simulink model "SFunBinToDes"  (R2019a)
settings: Solver=FixedStepDiscrete  StartTime=0.0  StopTime=10.0  RelTol=1e-3
settings Model: Creator=MY MIND  LastModifiedBy=MY MIND

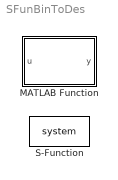
== system SFunBinToDes ==
  MATLAB Function : MATLAB Function  TreatAsAtomicUnit=on
  S-Function : S-Function  SFunctionDeploymentMode=off  EnableBusSupport=off

== matlab function SFunBinToDes/MATLAB Function ==
  data: u input; y output
function y = fcn(u)

y = u;
